simulink model "PI_AntiWindup"  (R2021a)
settings: Solver=FixedStepAuto  StartTime=0.0  StopTime=3  FixedStep=Ts  RelTol=1e-3
InitFcn:
  | run SetupParams.m
values from neighbouring files (symbols this model uses):
  Ka = 1 / Kp    (= 9.35278713056)    [SetupParams.m]
  Ki = 0.19812    [SetupParams.m]
  Kp = 0.10692    [SetupParams.m]
  omegaSlipBottomLim = -0.05 * omega_n    (= -15.7079632679)    [SetupParams.m]
  omegaSlipTopLim = 0.05 * omega_n    (= 15.7079632679)    [SetupParams.m]
libraries: cstblocks x1
settings Model: Creator=Charl  LastModifiedBy=Charl

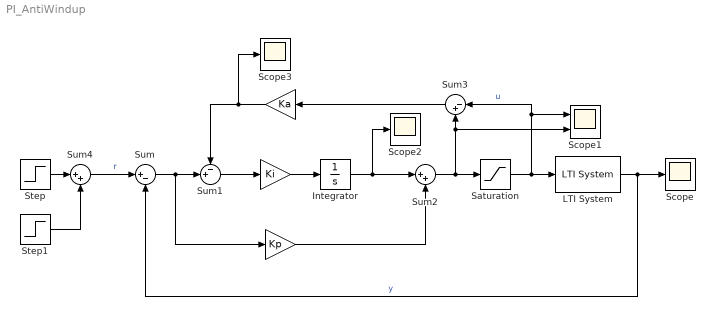
== system PI_AntiWindup ==
  " " : Gain  Gain=Ki
  "  " : Gain  Gain=Ka
  "   " : Gain  Gain=Kp
  Integrator : Integrator
  LTI System : cstblocks/LTI System  sys=G  IC=[]
  Saturation : Saturate  UpperLimit=omegaSlipTopLim  LowerLimit=omegaSlipBottomLim
  Scope : Scope
  Scope1 : Scope  NumInputPorts=2
  Scope2 : Scope
  Scope3 : Scope
  Step : Step  Time=0  After=100*2*pi  SampleTime=0
  Step1 : Step  Time=0.3  After=-100*2*pi  SampleTime=0
  Sum : Sum  Inputs=|+-
  Sum1 : Sum  Inputs=-+|
  Sum2 : Sum  Inputs=|++
  Sum3 : Sum  Inputs=|-+
  Sum4 : Sum  Inputs=|++
  wires:
  " "/1 -> Integrator/1
  LTI System/1 -> Sum/2, Scope/1  "y"
  Sum2/1 -> Saturation/1, Scope1/2, Sum3/2
  Integrator/1 -> Sum2/1, Scope2/1
  Sum3/1 -> "  "/1
  "  "/1 -> Scope3/1, Sum1/1
  Sum1/1 -> " "/1
  Sum/1 -> "   "/1, Sum1/2
  "   "/1 -> Sum2/2
  Saturation/1 -> LTI System/1, Sum3/1, Scope1/1  "u"
  Step/1 -> Sum4/1
  Sum4/1 -> Sum/1  "r"
  Step1/1 -> Sum4/2
